simulink model "pendule_inv_etu"  (R2022b)
settings: Solver=VariableStepAuto  StartTime=0.0  StopTime=10.0  RelTol=1e-3
values from neighbouring files (symbols this model uses):
  g = 9.81    [simu_pendule_inv_capteur_etu.m]    (also in simu_pendule_inv_echant_etu.m)
  K = [10 1]    [simu_pendule_inv_capteur_etu.m]    (also in simu_pendule_inv_echant_etu.m = [30 10])
  l = 10    [simu_pendule_inv_capteur_etu.m]    (also in simu_pendule_inv_echant_etu.m)
  ue = 0    [simu_pendule_inv_capteur_etu.m]    (also in simu_pendule_inv_echant_etu.m)
  x0 = [pi/20 0]'    [simu_pendule_inv_capteur_etu.m]    (also in simu_pendule_inv_echant_etu.m)
  xe = [0 0]'    [simu_pendule_inv_capteur_etu.m]    (also in simu_pendule_inv_echant_etu.m)
settings Model: Creator=felix  LastModifiedBy=felix

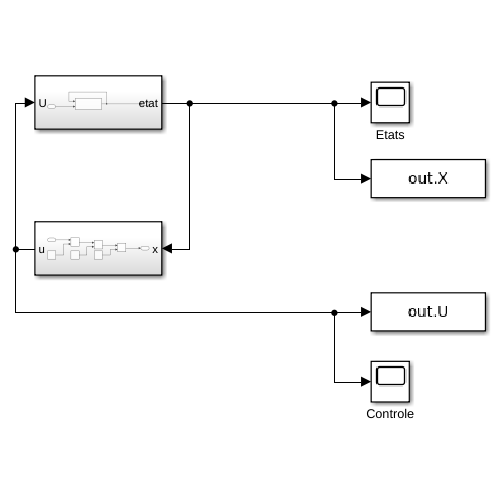
[thumbnail: Simulink's stored preview of the top-level diagram]
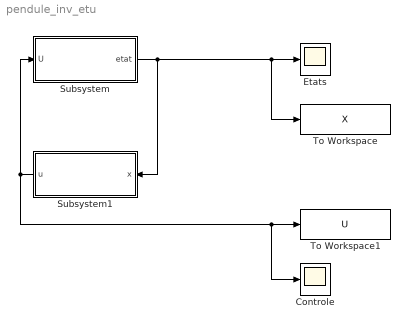
== system pendule_inv_etu ==
  Controle : Scope
  Etats : Scope
  Subsystem : Subsystem
  Subsystem1 : Subsystem
  To Workspace : ToWorkspace  VariableName=X  SaveFormat=Timeseries  SampleTime=-1
  To Workspace1 : ToWorkspace  VariableName=U  SaveFormat=Timeseries  SampleTime=-1
  wires:
  Subsystem/1(etat) -> Subsystem1/1(x), To Workspace/1, Etats/1
  Subsystem1/1(u) -> Subsystem/1(U), Controle/1, To Workspace1/1

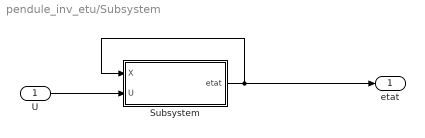
== system pendule_inv_etu/Subsystem ==
  U : Inport
  Subsystem : Subsystem
  etat : Outport
  wires:
  U/1 -> Subsystem/2(U)
  Subsystem/1(etat) -> Subsystem/1(X), etat/1

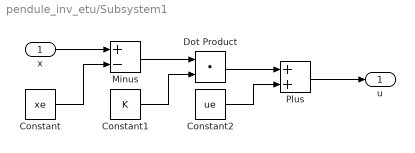
== system pendule_inv_etu/Subsystem1 ==
  x : Inport
  Constant : Constant  Value=xe
  Constant1 : Constant  Value=K
  Constant2 : Constant  Value=ue
  Dot Product : DotProduct  OutDataTypeStr=Inherit: Inherit via internal rule
  Minus : Sum  Inputs=+-
  Plus : Sum
  u : Outport
  wires:
  x/1 -> Minus/1
  Constant/1 -> Minus/2
  Minus/1 -> Dot Product/1
  Constant1/1 -> Dot Product/2
  Dot Product/1 -> Plus/1
  Constant2/1 -> Plus/2
  Plus/1 -> u/1

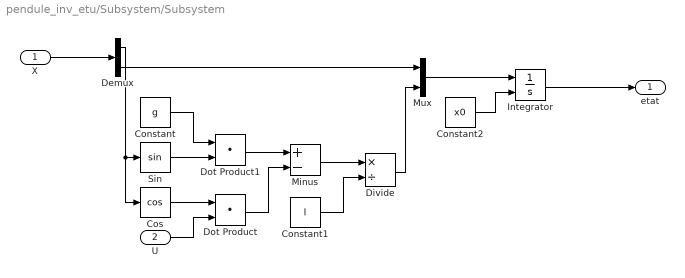
== system pendule_inv_etu/Subsystem/Subsystem ==
  X : Inport
  U : Inport  Port=2
  Constant : Constant  Value=g
  Constant1 : Constant  Value=l
  Constant2 : Constant  Value=x0
  Cos : Trigonometry  Operator=cos
  Demux : Demux  Outputs=2
  Divide : Product  Inputs=*/  RndMeth=Zero  SaturateOnIntegerOverflow=on
  Dot Product : DotProduct  OutDataTypeStr=Inherit: Inherit via internal rule
  Dot Product1 : DotProduct  OutDataTypeStr=Inherit: Inherit via internal rule
  Integrator : Integrator  InitialConditionSource=external
  Minus : Sum  Inputs=+-
  Mux : Mux  Inputs=2
  Sin : Trigonometry
  etat : Outport
  wires:
  X/1 -> Demux/1
  Mux/1 -> Integrator/1
  Demux/2 -> Mux/1
  Integrator/1 -> etat/1
  Demux/1 -> Cos/1, Sin/1
  Cos/1 -> Dot Product/1
  U/1 -> Dot Product/2
  Sin/1 -> Dot Product1/2
  Constant/1 -> Dot Product1/1
  Dot Product1/1 -> Minus/1
  Dot Product/1 -> Minus/2
  Minus/1 -> Divide/1
  Constant1/1 -> Divide/2
  Divide/1 -> Mux/2
  Constant2/1 -> Integrator/2
